simulink model "Hopf"  (R2022a)
settings: Solver=VariableStepAuto  StartTime=0.0  StopTime=30  RelTol=1e-3
settings Model: Creator=jandr  LastModifiedBy=jandr

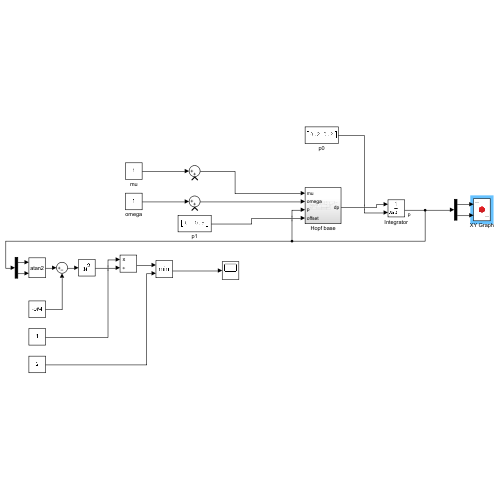
[thumbnail: Simulink's stored preview of the top-level diagram]
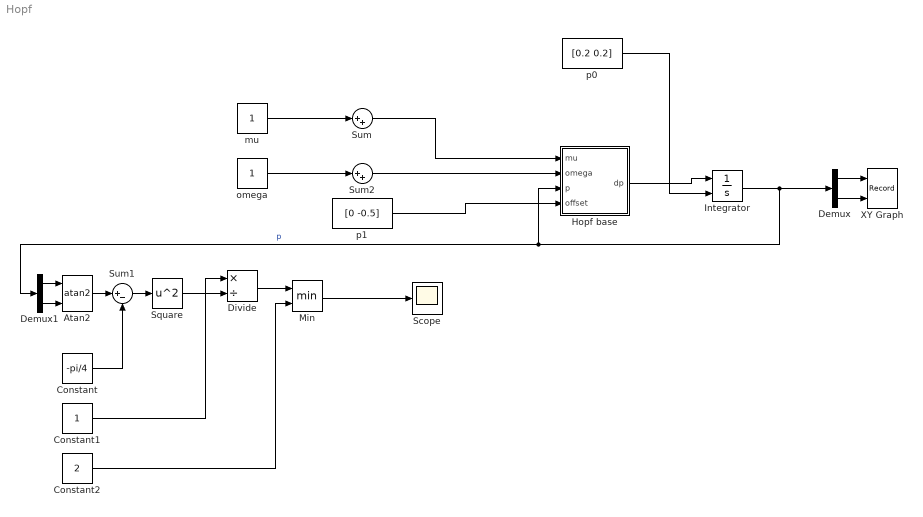
== system Hopf ==
  Atan2 : Trigonometry  Operator=atan2
  Constant : Constant  Value=-pi/4
  Constant1 : Constant
  Constant2 : Constant  Value=2
  Demux : Demux  Outputs=2
  Demux1 : Demux  Outputs=2
  Divide : Product  Inputs=*/
  Hopf base : Subsystem
  Integrator : Integrator  InitialConditionSource=external
  Min : MinMax  Inputs=2
  Scope : Scope
  Square : Math  Operator=square
  Sum : Sum  Inputs=|++
  Sum1 : Sum  Inputs=|+-
  Sum2 : Sum  Inputs=|++
  XY Graph : Record  FileSettingsInternal="{\"entries\":[{\"content\":{\"excelSettings\":{\"content\":{},\"type\":\"Streamout.ExcelSettings\"}},\"type\":\"Streamout.FileSettingStorage\",\"uuid\":\"5eb4f1f2-ebc8-462a-ba1b-b928507e6297\"}],\"packageUris\":[\"http://schema.mathworks.com/mf0/streamout_blocks/R2020a\"],\"version\":\"1.0\"}"  Layout=[1 1]  SignalsInternal="{\"entries\":[{\"content\":{\"signals\":[{\"content\":{\"blockPath\":[\"Hopf/XY Graph\"],\"channel\":[],\"dimensions\":[1],\"domain\":\"Hopf/XY Graph\",\"lineColor\":\"#a2142f\",\"plots\":[1],\"port\":1,\"sid\":[\"\"],\"signalID\":42,\"signalName\":\"Demux:1\"},\"type\":\"RecordBlkView.Signal\",\"uuid\":\"e1b8ff30-4f3e-4795-b73b-d6e48cd997b4\"},{\"content\":{\"blockPath\":[\"Hopf/XY Graph\"],\"channel\":[],\"dimensions\":[1],\"domain\":\"Hopf/XY Graph\",\"lineColor\":\"#139fff\",\"plots\":[1],\"port\":2,\"sid\":[\"\"],\"signalID\":46,\"signalName\":\"Demux:2\"},\"type\":\"RecordBlkView.Signal\",\"uuid\":\"638c7595-ee91-44e6-a4a9-ca95527487db\"}]},\"type\":\"RecordBlkView.InputSignals\",\"uuid\":\"5da901bb-c4d0-4abc-8976-59eeb3d8dafa\"}],\"packageUris\":[\"http://schema.mathworks.com/mf0/streamout_blocks/R2020a\"],\"version\":\"1.0\"}"  VisualizationBindings="{\"xyplotplugin\":{\"info\":[{\"series\":[{\"bindingParametersList\":[{\"parameter\":\"X-Axis\",\"signalID\":42,\"signalName\":\"Demux:1\"},{\"parameter\":\"Y-Axis\",\"signalID\":46,\"signalName\":\"Demux:2\"}],\"seriesID\":59289}],\"subplotID\":1}]}}"  CompatibilityTag=XY  st=-1
  mu : Constant
  omega : Constant
  p0 : Constant  Value=[0.2 0.2]
  p1 : Constant  Value=[0 -0.5]
  wires:
  p0/1 -> Integrator/2
  Hopf base/1(dp) -> Integrator/1
  Integrator/1 -> Demux/1, Hopf base/3(p), Demux1/1  "p"
  Demux/1 -> XY Graph/1
  Demux/2 -> XY Graph/2
  Sum2/1 -> Hopf base/2(omega)
  Sum/1 -> Hopf base/1(mu)
  mu/1 -> Sum/1
  Demux1/1 -> Atan2/1
  Demux1/2 -> Atan2/2
  Atan2/1 -> Sum1/1
  Sum1/1 -> Square/1
  Constant/1 -> Sum1/2
  Constant1/1 -> Divide/1
  Square/1 -> Divide/2
  Constant2/1 -> Min/2
  Divide/1 -> Min/1
  Min/1 -> Scope/1
  omega/1 -> Sum2/1
  p1/1 -> Hopf base/4(offset)

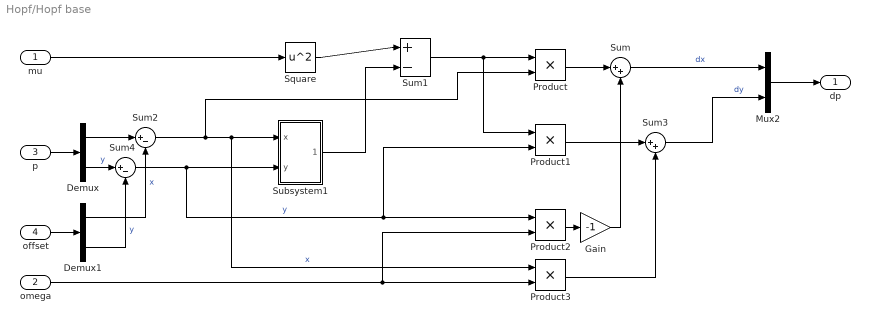
== system Hopf/Hopf base ==
  mu : Inport
  omega : Inport  Port=2
  p : Inport  Port=3
  offset : Inport  Port=4
  Demux : Demux  Outputs=2
  Demux1 : Demux  Outputs=2
  Gain : Gain  Gain=-1
  Mux2 : Mux  Inputs=2
  Product{,1..3} (4 alike) : Product
  Square : Math  Operator=square
  Subsystem1 : Subsystem
  Sum : Sum  Inputs=|++
  Sum1 : Sum  Inputs=|+-
  Sum2 : Sum  Inputs=|+-
  Sum3 : Sum  Inputs=|++
  Sum4 : Sum  Inputs=|+-
  dp : Outport
  wires:
  Gain/1 -> Sum/2
  Product1/1 -> Sum3/1
  Sum/1 -> Mux2/1  "dx"
  Subsystem1/1(rho2) -> Sum1/2
  Sum1/1 -> Product1/1, Product/1
  mu/1 -> Square/1
  Product/1 -> Sum/1
  Sum3/1 -> Mux2/2  "dy"
  Mux2/1 -> dp/1
  p/1 -> Demux/1
  Sum2/1 -> Product/2, Product3/1, Subsystem1/1(x)  "x"
  Sum4/1 -> Product2/1, Product1/2, Subsystem1/2(y)  "y"
  Square/1 -> Sum1/1
  Product2/1 -> Gain/1
  Product3/1 -> Sum3/2
  omega/1 -> Product2/2, Product3/2
  offset/1 -> Demux1/1
  Demux/1 -> Sum2/1
  Demux/2 -> Sum4/1  "y"
  Demux1/1 -> Sum2/2  "x"
  Demux1/2 -> Sum4/2  "y"

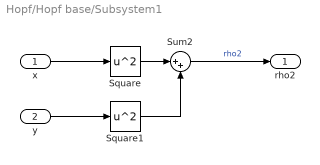
== system Hopf/Hopf base/Subsystem1 ==
  x : Inport
  y : Inport  Port=2
  Square : Math  Operator=square
  Square1 : Math  Operator=square
  Sum2 : Sum  Inputs=|++
  rho2 : Outport
  wires:
  Square/1 -> Sum2/1
  Sum2/1 -> rho2/1  "rho2"
  Square1/1 -> Sum2/2
  x/1 -> Square/1
  y/1 -> Square1/1
